simulink model "Lab_04_Task01"  (R2015a)
settings: Solver=ode45  StartTime=0.0  StopTime=10.0  RelTol=1e-3
libraries: cstblocks x4
settings Model: Creator=Amir  LastModifiedBy=Amir

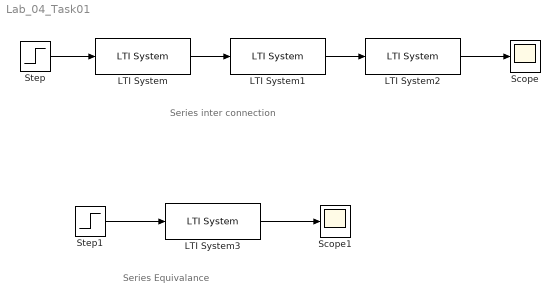
== system Lab_04_Task01 ==
  note: Series inter connection
  note: Series Equivalance
  LTI System : cstblocks/LTI System  sys=tf(1,[1 1])  IC=[]
  LTI System1 : cstblocks/LTI System  sys=tf(1,[1 3])  IC=[]
  LTI System2 : cstblocks/LTI System  sys=tf([1 3],[1 5])  IC=[]
  LTI System3 : cstblocks/LTI System  sys=tf([1 3],[1 9 23 15])  IC=[]
  Scope : Scope
  Scope1 : Scope
  Step : Step  SampleTime=0
  Step1 : Step  SampleTime=0
  wires:
  Step/1 -> LTI System/1
  LTI System/1 -> LTI System1/1
  LTI System1/1 -> LTI System2/1
  LTI System2/1 -> Scope/1
  Step1/1 -> LTI System3/1
  LTI System3/1 -> Scope1/1
